simulink model "labFinal_8"  (R2018b)
settings: Solver=FixedStepDiscrete  StartTime=0.0  StopTime=20.0  FixedStep=1  RelTol=1e-3
libraries: hdlsllib x127, simulink_extras x8
(part 1 of 4)
settings Model: Creator=mllax8  LastModifiedBy=mllax8

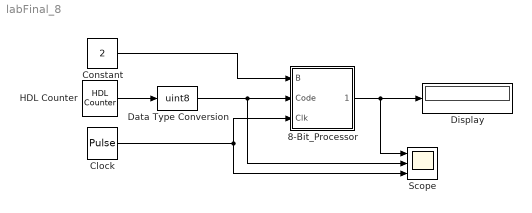
== system labFinal_8 ==
  8-Bit_Processor : Subsystem
  Clock : DiscretePulseGenerator
  Constant : Constant  Value=2  OutDataTypeStr=uint8  SampleTime=1
  Data Type Conversion : DataTypeConversion  OutDataTypeStr=uint8
  Display : Display
  HDL Counter : hdlsllib/Sources/HDL Counter  CountType=Free running  CountInit=0  CountStep=0.5  CountMax=25  CountFromType=Initial value  CountFrom=0  CountResetPort=off  CountLoadPort=off  CountEnbPort=off  CountDirPort=off  CountDataType=Unsigned  CountWordLen=3  CountFracLen=1  CountSampTime=1
      settings: SourceProductBaseCode=HD
  Scope : Scope  NumInputPorts=3
  wires:
  Constant/1 -> 8-Bit_Processor/1(B)
  Clock/1 -> 8-Bit_Processor/3(Clk), Scope/3
  8-Bit_Processor/1(Output) -> Scope/1, Display/1
  Data Type Conversion/1 -> Scope/2, 8-Bit_Processor/2(Code)
  HDL Counter/1 -> Data Type Conversion/1

== system labFinal_8/8-Bit_Processor ==
  B : Inport
  Code : Inport  Port=2
  Clk : Inport  Port=3
  8-bit 4-1 MUX : Subsystem
  8-bit_Adder : Subsystem
  8-bit_Bitwise_AND : Subsystem
  8-bit_Multiply : Subsystem
  8-bit_Register : Subsystem
  8-bit_Subtractor : Subsystem
  Data Type Conversion : DataTypeConversion  OutDataTypeStr=boolean
  Output : Outport
  wires:
  Clk/1 -> Data Type Conversion/1
  Data Type Conversion/1 -> 8-bit_Register/2(Clk)
  Code/1 -> 8-bit 4-1 MUX/1(S)
  8-bit_Adder/1(Sum) -> 8-bit 4-1 MUX/2(x0)
  8-bit_Multiply/1(Product) -> 8-bit 4-1 MUX/3(x1)
  8-bit_Subtractor/1(Diff) -> 8-bit 4-1 MUX/4(x2)
  8-bit_Bitwise_AND/1(Y) -> 8-bit 4-1 MUX/5(x3)
  8-bit_Register/1(Data_Out) -> 8-bit_Bitwise_AND/2(B), 8-bit_Subtractor/1(A), 8-bit_Multiply/2(B), 8-bit_Adder/2(B), Output/1
  8-bit 4-1 MUX/1(Out1) -> 8-bit_Register/1(Data_In)
  B/1 -> 8-bit_Subtractor/2(B), 8-bit_Bitwise_AND/1(A), 8-bit_Multiply/1(A), 8-bit_Adder/1(A)

== system labFinal_8/8-Bit_Processor/8-bit 4-1 MUX ==
  S : Inport
  x0 : Inport  Port=2
  x1 : Inport  Port=3
  x2 : Inport  Port=4
  x3 : Inport  Port=5
  4-1 MUX 2^0 : Subsystem
  4-1 MUX 2^1 : Subsystem
  4-1 MUX 2^2 : Subsystem
  4-1 MUX 2^3 : Subsystem
  4-1 MUX 2^4 : Subsystem
  4-1 MUX 2^5 : Subsystem
  4-1 MUX 2^6 : Subsystem
  4-1 MUX 2^7 : Subsystem
  Concat : Subsystem
  Slicer x0 : Subsystem
  Slicer x1 : Subsystem
  Slicer x2 : Subsystem
  Slicer x3 : Subsystem
  Out1 : Outport
  wires:
  x1/1 -> Slicer x1/1(uint8)
  x0/1 -> Slicer x0/1(uint8)
  4-1 MUX 2^0/1(Z) -> Concat/8(S 2^0)
  Slicer x2/2(B 2^6) -> 4-1 MUX 2^6/4(x2)
  4-1 MUX 2^2/1(Z) -> Concat/6(S 2^2)
  Slicer x2/7(B 2^1) -> 4-1 MUX 2^1/4(x2)
  4-1 MUX 2^5/1(Z) -> Concat/3(S 2^5)
  Slicer x1/3(B 2^5) -> 4-1 MUX 2^5/3(x1)
  Slicer x0/3(B 2^5) -> 4-1 MUX 2^5/2(x0)
  Slicer x3/8("B 2^0 ") -> 4-1 MUX 2^0/5(x3)
  4-1 MUX 2^4/1(Z) -> Concat/4(S 2^4)
  Slicer x2/8("B 2^0 ") -> 4-1 MUX 2^0/4(x2)
  Slicer x3/1(B 2^7) -> 4-1 MUX 2^7/5(x3)
  Slicer x2/4(B 2^4) -> 4-1 MUX 2^4/4(x2)
  Slicer x0/4(B 2^4) -> 4-1 MUX 2^4/2(x0)
  Slicer x1/8("B 2^0 ") -> 4-1 MUX 2^0/3(x1)
  Slicer x3/4(B 2^4) -> 4-1 MUX 2^4/5(x3)
  4-1 MUX 2^3/1(Z) -> Concat/5(S 2^3)
  Slicer x2/3(B 2^5) -> 4-1 MUX 2^5/4(x2)
  Slicer x3/6(B 2^2) -> 4-1 MUX 2^2/5(x3)
  x3/1 -> Slicer x3/1(uint8)
  Slicer x0/6(B 2^2) -> 4-1 MUX 2^2/2(x0)
  4-1 MUX 2^7/1(Z) -> Concat/1(S 2^7)
  Slicer x1/6(B 2^2) -> 4-1 MUX 2^2/3(x1)
  Slicer x3/2(B 2^6) -> 4-1 MUX 2^6/5(x3)
  Slicer x0/7(B 2^1) -> 4-1 MUX 2^1/2(x0)
  Slicer x2/6(B 2^2) -> 4-1 MUX 2^2/4(x2)
  Slicer x3/3(B 2^5) -> 4-1 MUX 2^5/5(x3)
  Slicer x1/7(B 2^1) -> 4-1 MUX 2^1/3(x1)
  x2/1 -> Slicer x2/1(uint8)
  Slicer x0/5(B 2^3) -> 4-1 MUX 2^3/2(x0)
  Slicer x1/5(B 2^3) -> 4-1 MUX 2^3/3(x1)
  Concat/1(unsign Int) -> Out1/1
  Slicer x2/1(B 2^7) -> 4-1 MUX 2^7/4(x2)
  Slicer x0/8("B 2^0 ") -> 4-1 MUX 2^0/2(x0)
  Slicer x2/5(B 2^3) -> 4-1 MUX 2^3/4(x2)
  4-1 MUX 2^1/1(Z) -> Concat/7(S 2^1)
  Slicer x3/7(B 2^1) -> 4-1 MUX 2^1/5(x3)
  4-1 MUX 2^6/1(Z) -> Concat/2(S 2^6)
  Slicer x1/2(B 2^6) -> 4-1 MUX 2^6/3(x1)
  Slicer x1/4(B 2^4) -> 4-1 MUX 2^4/3(x1)
  Slicer x0/2(B 2^6) -> 4-1 MUX 2^6/2(x0)
  Slicer x3/5(B 2^3) -> 4-1 MUX 2^3/5(x3)
  Slicer x1/1(B 2^7) -> 4-1 MUX 2^7/3(x1)
  S/1 -> 4-1 MUX 2^6/1(S), 4-1 MUX 2^5/1(S), 4-1 MUX 2^4/1(S), 4-1 MUX 2^3/1(S), 4-1 MUX 2^2/1(S), 4-1 MUX 2^0/1(S), 4-1 MUX 2^1/1(S), 4-1 MUX 2^7/1(S)
  Slicer x0/1(B 2^7) -> 4-1 MUX 2^7/2(x0)

== system labFinal_8/8-Bit_Processor/8-bit_Adder ==
  A : Inport  OutDataTypeStr=uint8
  B : Inport  Port=2  OutDataTypeStr=uint8
  2^0 : Subsystem
  2^1 : Subsystem
  2^2 : Subsystem
  2^3 : Subsystem
  2^4 : Subsystem
  2^5 : Subsystem
  2^6 : Subsystem
  2^7 : Subsystem
  Concat : Subsystem
  Constant : Constant  Value=0
  Overflow : Constant  Value=-1  OutDataTypeStr=double
  Slicer A : Subsystem
  Slicer B : Subsystem
  Switch : Switch  Criteria=u2 ~= 0
  Sum : Outport
  wires:
  Slicer B/8("B 2^0 ") -> 2^0/2(B)
  2^7/2(Sum) -> Concat/1(S 2^7)
  Slicer B/5(B 2^3) -> 2^3/2(B)
  2^3/2(Sum) -> Concat/5(S 2^3)
  2^5/1(Carry) -> 2^6/3(Carry In)
  Slicer B/4(B 2^4) -> 2^4/2(B)
  Constant/1 -> 2^0/3(Carry In)
  2^4/2(Sum) -> Concat/4(S 2^4)
  Slicer B/6(B 2^2) -> 2^2/2(B)
  2^6/2(Sum) -> Concat/2(S 2^6)
  Slicer A/7(A 2^1) -> 2^1/1(A)
  2^4/1(Carry) -> 2^5/3(Carry In)
  2^5/2(Sum) -> Concat/3(S 2^5)
  2^3/1(Carry) -> 2^4/3(Carry In)
  Slicer B/1(B 2^7) -> 2^7/2(B)
  Slicer A/1(A 2^7) -> 2^7/1(A)
  2^1/1(Carry) -> 2^2/3(Carry In)
  2^0/1(Carry) -> 2^1/3(Carry In)
  Slicer B/3(B 2^5) -> 2^5/2(B)
  Slicer A/8("A 2^0 ") -> 2^0/1(A)
  2^0/2(Sum) -> Concat/8(S 2^0)
  Slicer A/5(A 2^3) -> 2^3/1(A)
  2^2/1(Carry) -> 2^3/3(Carry In)
  Slicer B/7(B 2^1) -> 2^1/2(B)
  Slicer A/4(A 2^4) -> 2^4/1(A)
  2^2/2(Sum) -> Concat/6(S 2^2)
  2^6/1(Carry) -> 2^7/3(Carry In)
  B/1 -> Slicer B/1(uint8)
  Slicer A/2(A 2^6) -> 2^6/1(A)
  2^1/2(Sum) -> Concat/7(S 2^1)
  Slicer A/3(A 2^5) -> 2^5/1(A)
  Slicer B/2(B 2^6) -> 2^6/2(B)
  2^7/1(Carry) -> Switch/2
  Slicer A/6(A 2^2) -> 2^2/1(A)
  A/1 -> Slicer A/1(uint8)
  Overflow/1 -> Switch/1
  Switch/1 -> Sum/1
  Concat/1(unsign Int) -> Switch/3

== system labFinal_8/8-Bit_Processor/8-bit_Bitwise_AND ==
  A : Inport  OutDataTypeStr=uint8
  B : Inport  Port=2  OutDataTypeStr=uint8
  Concat : Subsystem
  Logical Operator{,1..7} (8 alike) : Logic  AllPortsSameDT=off  OutDataTypeStr=boolean
  Slicer A : Subsystem
  Slicer B : Subsystem
  Y : Outport
  wires:
  B/1 -> Slicer B/1(uint8)
  A/1 -> Slicer A/1(uint8)
  Logical Operator/1 -> Concat/8(S 2^0)
  Slicer B/8("B 2^0 ") -> Logical Operator/2
  Slicer A/8("A 2^0 ") -> Logical Operator/1
  Logical Operator1/1 -> Concat/7(S 2^1)
  Logical Operator2/1 -> Concat/6(S 2^2)
  Logical Operator4/1 -> Concat/4(S 2^4)
  Logical Operator3/1 -> Concat/5(S 2^3)
  Logical Operator5/1 -> Concat/3(S 2^5)
  Logical Operator6/1 -> Concat/2(S 2^6)
  Logical Operator7/1 -> Concat/1(S 2^7)
  Slicer B/7(B 2^1) -> Logical Operator1/2
  Slicer B/6(B 2^2) -> Logical Operator2/2
  Slicer B/5(B 2^3) -> Logical Operator3/2
  Slicer B/4(B 2^4) -> Logical Operator4/2
  Slicer B/3(B 2^5) -> Logical Operator5/2
  Slicer B/2(B 2^6) -> Logical Operator6/2
  Slicer B/1(B 2^7) -> Logical Operator7/2
  Slicer A/7(A 2^1) -> Logical Operator1/1
  Slicer A/6(A 2^2) -> Logical Operator2/1
  Slicer A/5(A 2^3) -> Logical Operator3/1
  Slicer A/4(A 2^4) -> Logical Operator4/1
  Slicer A/3(A 2^5) -> Logical Operator5/1
  Slicer A/2(A 2^6) -> Logical Operator6/1
  Slicer A/1(A 2^7) -> Logical Operator7/1
  Concat/1(unsign Int) -> Y/1

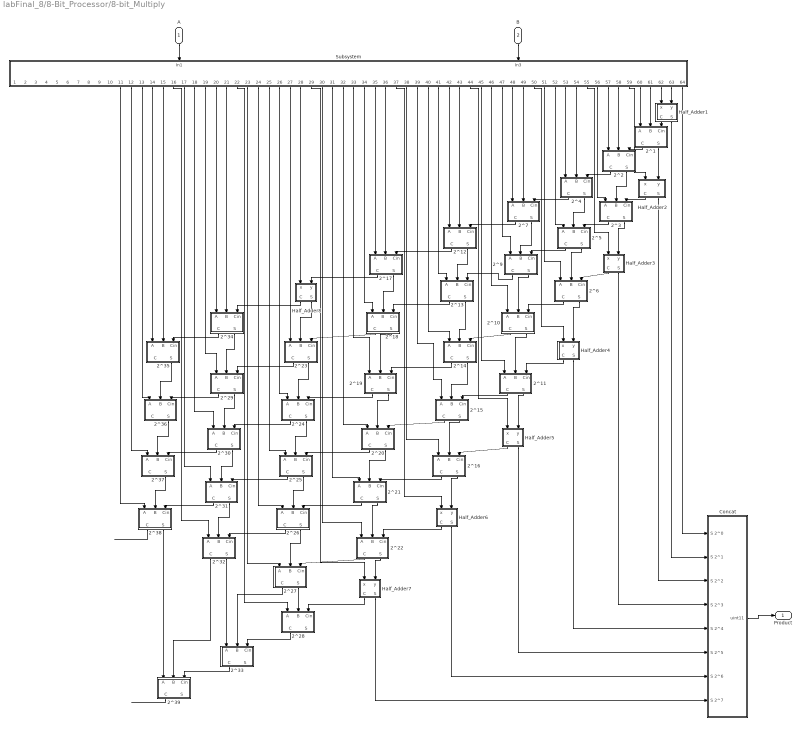
== system labFinal_8/8-Bit_Processor/8-bit_Multiply ==
  A : Inport  OutDataTypeStr=uint8
  B : Inport  Port=2  OutDataTypeStr=uint8
  2^1 : Subsystem
  2^10 : Subsystem
  2^11 : Subsystem
  2^12 : Subsystem
  2^13 : Subsystem
  2^14 : Subsystem
  2^15 : Subsystem
  2^16 : Subsystem
  2^17 : Subsystem
  2^18 : Subsystem
  2^19 : Subsystem
  2^2 : Subsystem
  2^20 : Subsystem
  2^21 : Subsystem
  2^22 : Subsystem
  2^23 : Subsystem
  2^24 : Subsystem
  2^25 : Subsystem
  2^26 : Subsystem
  2^27 : Subsystem
  2^28 : Subsystem
  2^29 : Subsystem
  2^3 : Subsystem
  2^30 : Subsystem
  2^31 : Subsystem
  2^32 : Subsystem
  2^33 : Subsystem
  2^34 : Subsystem
  2^35 : Subsystem
  2^36 : Subsystem
  2^37 : Subsystem
  2^38 : Subsystem
  2^39 : Subsystem
  2^4 : Subsystem
  2^5 : Subsystem
  2^6 : Subsystem
  2^7 : Subsystem
  2^9 : Subsystem
  Concat : Subsystem
  Half_Adder1 : Subsystem
  Half_Adder2 : Subsystem
  Half_Adder3 : Subsystem
  Half_Adder4 : Subsystem
  Half_Adder5 : Subsystem
  Half_Adder6 : Subsystem
  Half_Adder7 : Subsystem
  Half_Adder8 : Subsystem
  Subsystem : Subsystem
  Product : Outport
  wires:
  A/1 -> Subsystem/1(In1)
  B/1 -> Subsystem/2(In3)
  Subsystem/63(A0B1) -> Half_Adder1/2(y)
  Subsystem/62(A1B0) -> Half_Adder1/1(x)
  Half_Adder1/1(C) -> 2^1/3(Cin)
  Subsystem/61(A1B1) -> 2^1/2(B)
  Subsystem/60(A0B2) -> 2^1/1(A)
  Subsystem/59(A2B0) -> Half_Adder2/1(x)
  2^1/2(S) -> Half_Adder2/2(y)
  2^1/1(C) -> 2^2/3(Cin)
  Subsystem/58(A0B3) -> 2^2/2(B)
  Subsystem/57(A1B2) -> 2^2/1(A)
  Half_Adder2/1(C) -> 2^3/3(Cin)
  2^2/2(S) -> 2^3/2(B)
  Subsystem/56(A2B1) -> 2^3/1(A)
  2^3/1(C) -> 2^5/3(Cin)
  Subsystem/55(A3B0) -> Half_Adder3/1(x)
  2^3/2(S) -> Half_Adder3/2(y)
  Subsystem/54(A0B4) -> 2^4/2(B)
  Subsystem/53(A1B3) -> 2^4/1(A)
  2^2/1(C) -> 2^4/3(Cin)
  2^4/1(C) -> 2^7/3(Cin)
  2^4/2(S) -> 2^5/2(B)
  Subsystem/52(A2B2) -> 2^5/1(A)
  2^5/1(C) -> 2^9/3(Cin)
  Half_Adder3/1(C) -> 2^6/3(Cin)
  2^5/2(S) -> 2^6/2(B)
  Subsystem/51(A3B1) -> 2^6/1(A)
  2^6/1(C) -> 2^10/3(Cin)
  2^6/2(S) -> Half_Adder4/2(y)
  Subsystem/50(A4B0) -> Half_Adder4/1(x)
  Half_Adder4/1(C) -> 2^11/3(Cin)
  Subsystem/49(A0B5) -> 2^7/2(B)
  Subsystem/48(A1B4) -> 2^7/1(A)
  Subsystem/47(A2B3) -> 2^9/1(A)
  2^9/2(S) -> 2^10/2(B)
  2^9/1(C) -> 2^13/3(Cin)
  2^7/2(S) -> 2^9/2(B)
  2^7/1(C) -> 2^12/3(Cin)
  Subsystem/46(A3B2) -> 2^10/1(A)
  2^10/1(C) -> 2^14/3(Cin)
  2^10/2(S) -> 2^11/2(B)
  Half_Adder3/2(S) -> Concat/4(S 2^3)
  Half_Adder4/2(S) -> Concat/5(S 2^4)
  2^11/1(C) -> 2^15/3(Cin)
  Subsystem/44(A5B0) -> Half_Adder5/1(x)
  2^11/2(S) -> Half_Adder5/2(y)
  Half_Adder5/2(S) -> Concat/6(S 2^5)
  Half_Adder5/1(C) -> 2^16/3(Cin)
  Subsystem/43(A0B6) -> 2^12/2(B)
  Subsystem/42(A1B5) -> 2^12/1(A)
  2^12/2(S) -> 2^13/2(B)
  Subsystem/41(A2B4) -> 2^13/1(A)
  Subsystem/45(A4B1) -> 2^11/1(A)
  2^13/1(C) -> 2^18/3(Cin)
  2^13/2(S) -> 2^14/2(B)
  Subsystem/40(A3B3) -> 2^14/1(A)
  2^14/2(S) -> 2^15/2(B)
  Subsystem/39(A4B2) -> 2^15/1(A)
  2^15/2(S) -> 2^16/2(B)
  Subsystem/38(A5B1) -> 2^16/1(A)
  2^15/1(C) -> 2^20/3(Cin)
  2^16/1(C) -> 2^21/3(Cin)
  Subsystem/37(A6B0) -> Half_Adder6/1(x)
  2^16/2(S) -> Half_Adder6/2(y)
  Half_Adder6/2(S) -> Concat/7(S 2^6)
  Half_Adder6/1(C) -> 2^22/3(Cin)
  2^17/1(C) -> Half_Adder8/2(y)
  2^12/1(C) -> 2^17/3(Cin)
  2^18/2(S) -> 2^19/2(B)
  2^21/1(C) -> 2^26/3(Cin)
  Subsystem/33(A3B4) -> 2^19/1(A)
  2^19/2(S) -> 2^20/2(B)
  Subsystem/34(A2B5) -> 2^18/1(A)
  Subsystem/32(A4B3) -> 2^20/1(A)
  2^20/2(S) -> 2^21/2(B)
  2^18/1(C) -> 2^23/3(Cin)
  Subsystem/31(A5B2) -> 2^21/1(A)
  2^17/2(S) -> 2^18/2(B)
  Subsystem/36(A0B7) -> 2^17/2(B)
  Subsystem/35(A1B6) -> 2^17/1(A)
  2^14/1(C) -> 2^19/3(Cin)
  2^21/2(S) -> 2^22/2(B)
  Subsystem/30(A6B1) -> 2^22/1(A)
  Subsystem/64(A0B0) -> Concat/1(S 2^0)
  Half_Adder2/2(S) -> Concat/3(S 2^2)
  2^22/2(S) -> Half_Adder7/2(y)
  Subsystem/29(A7B0) -> Half_Adder7/1(x)
  Subsystem/28(A1B7) -> Half_Adder8/1(x)
  Subsystem/27(A2B6) -> 2^23/1(A)
  Half_Adder8/2(S) -> 2^23/2(B)
  Half_Adder8/1(C) -> 2^34/3(Cin)
  2^19/1(C) -> 2^24/3(Cin)
  2^23/2(S) -> 2^24/2(B)
  Subsystem/26(A3B5) -> 2^24/1(A)
  2^20/1(C) -> 2^25/3(Cin)
  2^24/2(S) -> 2^25/2(B)
  Subsystem/25(A4B4) -> 2^25/1(A)
  2^24/1(C) -> 2^30/3(Cin)
  2^25/2(S) -> 2^26/2(B)
  2^25/1(C) -> 2^31/3(Cin)
  2^22/1(C) -> 2^27/3(Cin)
  Subsystem/24(A5B3) -> 2^26/1(A)
  Subsystem/23(A6B2) -> 2^27/1(A)
  Subsystem/22(A7B1) -> 2^28/1(A)
  2^26/2(S) -> 2^27/2(B)
  Half_Adder7/1(C) -> 2^28/3(Cin)
  2^27/2(S) -> 2^28/2(B)
  2^26/1(C) -> 2^32/3(Cin)
  Half_Adder7/2(S) -> Concat/8(S 2^7)
  2^28/1(C) -> 2^33/3(Cin)
  2^29/2(S) -> 2^30/2(B)
  2^30/2(S) -> 2^31/2(B)
  2^31/2(S) -> 2^32/2(B)
  Subsystem/21(A2B7) -> 2^34/2(B)
  Subsystem/20(A3B6) -> 2^34/1(A)
  2^23/1(C) -> 2^29/3(Cin)
  2^34/2(S) -> 2^29/2(B)
  Subsystem/19(A4B5) -> 2^29/1(A)
  Subsystem/18(A5B4) -> 2^30/1(A)
  Subsystem/17(A6B3) -> 2^31/1(A)
  Subsystem/16(A7B2) -> 2^32/1(A)
  2^32/2(S) -> 2^33/1(A)
  2^27/1(C) -> 2^33/2(B)
  2^32/1(C) -> 2^39/2(B)
  2^33/1(C) -> 2^39/3(Cin)
  2^34/1(C) -> 2^35/3(Cin)
  Subsystem/15(A3B7) -> 2^35/2(B)
  Subsystem/14(A4B6) -> 2^35/1(A)
  2^35/2(S) -> 2^36/2(B)
  2^29/1(C) -> 2^36/3(Cin)
  2^30/1(C) -> 2^37/3(Cin)
  2^36/2(S) -> 2^37/2(B)
  Subsystem/13(A5B5) -> 2^36/1(A)
  Subsystem/12(A6B4) -> 2^37/1(A)
  Subsystem/11(A7B3) -> 2^38/1(A)
  2^31/1(C) -> 2^38/3(Cin)
  2^37/2(S) -> 2^38/2(B)
  2^38/2(S) -> 2^39/1(A)
  2^38/1(C) -> ?
  2^39/1(C) -> ?
  Half_Adder1/2(S) -> Concat/2(S 2^1)
  Concat/1(uint11) -> Product/1

== system labFinal_8/8-Bit_Processor/8-bit_Register ==
  Data_In : Inport  OutDataTypeStr=uint8
  Clk : Inport  Port=2
  Concat : Subsystem
  Constant : Constant  OutDataTypeStr=boolean  SampleTime=1
  D Flip-Flop{,1..7} (8 alike) : simulink_extras/Flip Flops/D Flip-Flop
      settings: SourceProductName=Simulink
  Slicer A : Subsystem
  Data_Out : Outport
  wires:
  Data_In/1 -> Slicer A/1(uint8)
  Constant/1 -> D Flip-Flop7/3, D Flip-Flop6/3, D Flip-Flop5/3, D Flip-Flop4/3, D Flip-Flop3/3, D Flip-Flop2/3, D Flip-Flop1/3, D Flip-Flop/3
  Clk/1 -> D Flip-Flop7/2, D Flip-Flop6/2, D Flip-Flop5/2, D Flip-Flop4/2, D Flip-Flop3/2, D Flip-Flop2/2, D Flip-Flop1/2, D Flip-Flop/2
  D Flip-Flop/1 -> Concat/8(S 2^0)
  Slicer A/1(A 2^7) -> D Flip-Flop7/1
  Slicer A/2(A 2^6) -> D Flip-Flop6/1
  Slicer A/3(A 2^5) -> D Flip-Flop5/1
  Slicer A/4(A 2^4) -> D Flip-Flop4/1
  Slicer A/5(A 2^3) -> D Flip-Flop3/1
  Slicer A/6(A 2^2) -> D Flip-Flop2/1
  Slicer A/7(A 2^1) -> D Flip-Flop1/1
  Slicer A/8("A 2^0 ") -> D Flip-Flop/1
  D Flip-Flop1/1 -> Concat/7(S 2^1)
  D Flip-Flop7/1 -> Concat/1(S 2^7)
  D Flip-Flop6/1 -> Concat/2(S 2^6)
  D Flip-Flop5/1 -> Concat/3(S 2^5)
  D Flip-Flop4/1 -> Concat/4(S 2^4)
  D Flip-Flop3/1 -> Concat/5(S 2^3)
  D Flip-Flop2/1 -> Concat/6(S 2^2)
  Concat/1(unsign Int) -> Data_Out/1

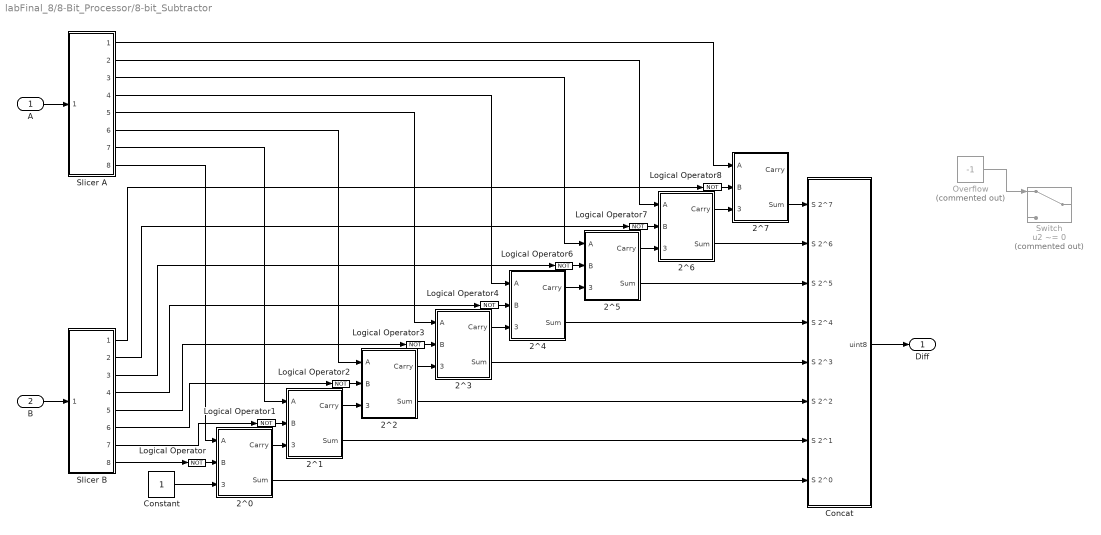
== system labFinal_8/8-Bit_Processor/8-bit_Subtractor ==
  A : Inport  OutDataTypeStr=uint8
  B : Inport  Port=2  OutDataTypeStr=uint8
  2^0 : Subsystem
  2^1 : Subsystem
  2^2 : Subsystem
  2^3 : Subsystem
  2^4 : Subsystem
  2^5 : Subsystem
  2^6 : Subsystem
  2^7 : Subsystem
  Concat : Subsystem
  Constant : Constant  SampleTime=1
  Logical Operator{,1..4,6..8} (8 alike) : Logic  Operator=NOT  AllPortsSameDT=off  OutDataTypeStr=boolean
  Overflow : Constant  Commented=on  Value=-1  OutDataTypeStr=double
  Slicer A : Subsystem
  Slicer B : Subsystem
  Switch : Switch  Commented=on  Criteria=u2 ~= 0
  Diff : Outport
  wires:
  2^7/2(Sum) -> Concat/1(S 2^7)
  Slicer B/5(B 2^3) -> Logical Operator3/1
  2^3/2(Sum) -> Concat/5(S 2^3)
  2^5/1(Carry) -> 2^6/3(Carry In)
  Slicer B/4(B 2^4) -> Logical Operator4/1
  Constant/1 -> 2^0/3(Carry In)
  2^4/2(Sum) -> Concat/4(S 2^4)
  Slicer B/6(B 2^2) -> Logical Operator2/1
  2^6/2(Sum) -> Concat/2(S 2^6)
  Slicer A/7(A 2^1) -> 2^1/1(A)
  2^4/1(Carry) -> 2^5/3(Carry In)
  2^5/2(Sum) -> Concat/3(S 2^5)
  2^3/1(Carry) -> 2^4/3(Carry In)
  Slicer B/1(B 2^7) -> Logical Operator8/1
  Slicer A/1(A 2^7) -> 2^7/1(A)
  2^1/1(Carry) -> 2^2/3(Carry In)
  2^0/1(Carry) -> 2^1/3(Carry In)
  Slicer B/3(B 2^5) -> Logical Operator6/1
  Slicer A/8("A 2^0 ") -> 2^0/1(A)
  2^0/2(Sum) -> Concat/8(S 2^0)
  Slicer A/5(A 2^3) -> 2^3/1(A)
  2^2/1(Carry) -> 2^3/3(Carry In)
  Slicer B/7(B 2^1) -> Logical Operator1/1
  Slicer A/4(A 2^4) -> 2^4/1(A)
  2^2/2(Sum) -> Concat/6(S 2^2)
  2^6/1(Carry) -> 2^7/3(Carry In)
  B/1 -> Slicer B/1(uint8)
  Slicer A/2(A 2^6) -> 2^6/1(A)
  2^1/2(Sum) -> Concat/7(S 2^1)
  Slicer A/3(A 2^5) -> 2^5/1(A)
  Slicer B/2(B 2^6) -> Logical Operator7/1
  Slicer A/6(A 2^2) -> 2^2/1(A)
  A/1 -> Slicer A/1(uint8)
  Overflow/1 -> Switch/1
  Logical Operator/1 -> 2^0/2(B)
  Slicer B/8("B 2^0 ") -> Logical Operator/1
  Logical Operator1/1 -> 2^1/2(B)
  Logical Operator2/1 -> 2^2/2(B)
  Logical Operator3/1 -> 2^3/2(B)
  Logical Operator4/1 -> 2^4/2(B)
  Logical Operator6/1 -> 2^5/2(B)
  Logical Operator7/1 -> 2^6/2(B)
  Logical Operator8/1 -> 2^7/2(B)
  Concat/1(uint8) -> Diff/1

== system labFinal_8/8-Bit_Processor/8-bit 4-1 MUX/4-1 MUX 2^0 ==
  S : Inport  OutDataTypeStr=uint8
  x0 : Inport  Port=2  OutDataTypeStr=boolean
  x1 : Inport  Port=3  OutDataTypeStr=boolean
  x2 : Inport  Port=4  OutDataTypeStr=boolean
  x3 : Inport  Port=5  OutDataTypeStr=boolean
  2-1 MUX1 : Subsystem
  2-1 MUX2 : Subsystem
  2-1 MUX3 : Subsystem
  Slicer Code : Subsystem
  Z : Outport
  wires:
  Slicer Code/2("S 2^0 ") -> 2-1 MUX3/1(S), 2-1 MUX1/1(S)
  x0/1 -> 2-1 MUX3/2(I0)
  x1/1 -> 2-1 MUX3/3(I1)
  x2/1 -> 2-1 MUX1/2(I0)
  x3/1 -> 2-1 MUX1/3(I1)
  2-1 MUX3/1(Z) -> 2-1 MUX2/2(I0)
  2-1 MUX1/1(Z) -> 2-1 MUX2/3(I1)
  2-1 MUX2/1(Z) -> Z/1
  S/1 -> Slicer Code/1(uint8)
  Slicer Code/1(S 2^1) -> 2-1 MUX2/1(S)

== system labFinal_8/8-Bit_Processor/8-bit 4-1 MUX/4-1 MUX 2^1 ==
  S : Inport  OutDataTypeStr=uint8
  x0 : Inport  Port=2  OutDataTypeStr=boolean
  x1 : Inport  Port=3  OutDataTypeStr=boolean
  x2 : Inport  Port=4  OutDataTypeStr=boolean
  x3 : Inport  Port=5  OutDataTypeStr=boolean
  2-1 MUX1 : Subsystem
  2-1 MUX2 : Subsystem
  2-1 MUX3 : Subsystem
  Slicer Code : Subsystem
  Z : Outport
  wires:
  Slicer Code/2("S 2^0 ") -> 2-1 MUX3/1(S), 2-1 MUX1/1(S)
  x0/1 -> 2-1 MUX3/2(I0)
  x1/1 -> 2-1 MUX3/3(I1)
  x2/1 -> 2-1 MUX1/2(I0)
  x3/1 -> 2-1 MUX1/3(I1)
  2-1 MUX3/1(Z) -> 2-1 MUX2/2(I0)
  2-1 MUX1/1(Z) -> 2-1 MUX2/3(I1)
  2-1 MUX2/1(Z) -> Z/1
  S/1 -> Slicer Code/1(uint8)
  Slicer Code/1(S 2^1) -> 2-1 MUX2/1(S)

== system labFinal_8/8-Bit_Processor/8-bit 4-1 MUX/4-1 MUX 2^2 ==
  S : Inport  OutDataTypeStr=uint8
  x0 : Inport  Port=2  OutDataTypeStr=boolean
  x1 : Inport  Port=3  OutDataTypeStr=boolean
  x2 : Inport  Port=4  OutDataTypeStr=boolean
  x3 : Inport  Port=5  OutDataTypeStr=boolean
  2-1 MUX1 : Subsystem
  2-1 MUX2 : Subsystem
  2-1 MUX3 : Subsystem
  Slicer Code : Subsystem
  Z : Outport
  wires:
  Slicer Code/2("S 2^0 ") -> 2-1 MUX3/1(S), 2-1 MUX1/1(S)
  x0/1 -> 2-1 MUX3/2(I0)
  x1/1 -> 2-1 MUX3/3(I1)
  x2/1 -> 2-1 MUX1/2(I0)
  x3/1 -> 2-1 MUX1/3(I1)
  2-1 MUX3/1(Z) -> 2-1 MUX2/2(I0)
  2-1 MUX1/1(Z) -> 2-1 MUX2/3(I1)
  2-1 MUX2/1(Z) -> Z/1
  S/1 -> Slicer Code/1(uint8)
  Slicer Code/1(S 2^1) -> 2-1 MUX2/1(S)

== system labFinal_8/8-Bit_Processor/8-bit 4-1 MUX/4-1 MUX 2^3 ==
  S : Inport  OutDataTypeStr=uint8
  x0 : Inport  Port=2  OutDataTypeStr=boolean
  x1 : Inport  Port=3  OutDataTypeStr=boolean
  x2 : Inport  Port=4  OutDataTypeStr=boolean
  x3 : Inport  Port=5  OutDataTypeStr=boolean
  2-1 MUX1 : Subsystem
  2-1 MUX2 : Subsystem
  2-1 MUX3 : Subsystem
  Slicer Code : Subsystem
  Z : Outport
  wires:
  Slicer Code/2("S 2^0 ") -> 2-1 MUX3/1(S), 2-1 MUX1/1(S)
  x0/1 -> 2-1 MUX3/2(I0)
  x1/1 -> 2-1 MUX3/3(I1)
  x2/1 -> 2-1 MUX1/2(I0)
  x3/1 -> 2-1 MUX1/3(I1)
  2-1 MUX3/1(Z) -> 2-1 MUX2/2(I0)
  2-1 MUX1/1(Z) -> 2-1 MUX2/3(I1)
  2-1 MUX2/1(Z) -> Z/1
  S/1 -> Slicer Code/1(uint8)
  Slicer Code/1(S 2^1) -> 2-1 MUX2/1(S)

== system labFinal_8/8-Bit_Processor/8-bit 4-1 MUX/4-1 MUX 2^4 ==
  S : Inport  OutDataTypeStr=uint8
  x0 : Inport  Port=2  OutDataTypeStr=boolean
  x1 : Inport  Port=3  OutDataTypeStr=boolean
  x2 : Inport  Port=4  OutDataTypeStr=boolean
  x3 : Inport  Port=5  OutDataTypeStr=boolean
  2-1 MUX1 : Subsystem
  2-1 MUX2 : Subsystem
  2-1 MUX3 : Subsystem
  Slicer Code : Subsystem
  Z : Outport
  wires:
  Slicer Code/2("S 2^0 ") -> 2-1 MUX3/1(S), 2-1 MUX1/1(S)
  x0/1 -> 2-1 MUX3/2(I0)
  x1/1 -> 2-1 MUX3/3(I1)
  x2/1 -> 2-1 MUX1/2(I0)
  x3/1 -> 2-1 MUX1/3(I1)
  2-1 MUX3/1(Z) -> 2-1 MUX2/2(I0)
  2-1 MUX1/1(Z) -> 2-1 MUX2/3(I1)
  2-1 MUX2/1(Z) -> Z/1
  S/1 -> Slicer Code/1(uint8)
  Slicer Code/1(S 2^1) -> 2-1 MUX2/1(S)

== system labFinal_8/8-Bit_Processor/8-bit 4-1 MUX/4-1 MUX 2^5 ==
  S : Inport  OutDataTypeStr=uint8
  x0 : Inport  Port=2  OutDataTypeStr=boolean
  x1 : Inport  Port=3  OutDataTypeStr=boolean
  x2 : Inport  Port=4  OutDataTypeStr=boolean
  x3 : Inport  Port=5  OutDataTypeStr=boolean
  2-1 MUX1 : Subsystem
  2-1 MUX2 : Subsystem
  2-1 MUX3 : Subsystem
  Slicer Code : Subsystem
  Z : Outport
  wires:
  Slicer Code/2("S 2^0 ") -> 2-1 MUX3/1(S), 2-1 MUX1/1(S)
  x0/1 -> 2-1 MUX3/2(I0)
  x1/1 -> 2-1 MUX3/3(I1)
  x2/1 -> 2-1 MUX1/2(I0)
  x3/1 -> 2-1 MUX1/3(I1)
  2-1 MUX3/1(Z) -> 2-1 MUX2/2(I0)
  2-1 MUX1/1(Z) -> 2-1 MUX2/3(I1)
  2-1 MUX2/1(Z) -> Z/1
  S/1 -> Slicer Code/1(uint8)
  Slicer Code/1(S 2^1) -> 2-1 MUX2/1(S)

== system labFinal_8/8-Bit_Processor/8-bit 4-1 MUX/4-1 MUX 2^6 ==
  S : Inport  OutDataTypeStr=uint8
  x0 : Inport  Port=2  OutDataTypeStr=boolean
  x1 : Inport  Port=3  OutDataTypeStr=boolean
  x2 : Inport  Port=4  OutDataTypeStr=boolean
  x3 : Inport  Port=5  OutDataTypeStr=boolean
  2-1 MUX1 : Subsystem
  2-1 MUX2 : Subsystem
  2-1 MUX3 : Subsystem
  Slicer Code : Subsystem
  Z : Outport
  wires:
  Slicer Code/2("S 2^0 ") -> 2-1 MUX3/1(S), 2-1 MUX1/1(S)
  x0/1 -> 2-1 MUX3/2(I0)
  x1/1 -> 2-1 MUX3/3(I1)
  x2/1 -> 2-1 MUX1/2(I0)
  x3/1 -> 2-1 MUX1/3(I1)
  2-1 MUX3/1(Z) -> 2-1 MUX2/2(I0)
  2-1 MUX1/1(Z) -> 2-1 MUX2/3(I1)
  2-1 MUX2/1(Z) -> Z/1
  S/1 -> Slicer Code/1(uint8)
  Slicer Code/1(S 2^1) -> 2-1 MUX2/1(S)

== system labFinal_8/8-Bit_Processor/8-bit 4-1 MUX/4-1 MUX 2^7 ==
  S : Inport  OutDataTypeStr=uint8
  x0 : Inport  Port=2  OutDataTypeStr=boolean
  x1 : Inport  Port=3  OutDataTypeStr=boolean
  x2 : Inport  Port=4  OutDataTypeStr=boolean
  x3 : Inport  Port=5  OutDataTypeStr=boolean
  2-1 MUX1 : Subsystem
  2-1 MUX2 : Subsystem
  2-1 MUX3 : Subsystem
  Slicer Code : Subsystem
  Z : Outport
  wires:
  Slicer Code/2("S 2^0 ") -> 2-1 MUX3/1(S), 2-1 MUX1/1(S)
  x0/1 -> 2-1 MUX3/2(I0)
  x1/1 -> 2-1 MUX3/3(I1)
  x2/1 -> 2-1 MUX1/2(I0)
  x3/1 -> 2-1 MUX1/3(I1)
  2-1 MUX3/1(Z) -> 2-1 MUX2/2(I0)
  2-1 MUX1/1(Z) -> 2-1 MUX2/3(I1)
  2-1 MUX2/1(Z) -> Z/1
  S/1 -> Slicer Code/1(uint8)
  Slicer Code/1(S 2^1) -> 2-1 MUX2/1(S)

== system labFinal_8/8-Bit_Processor/8-bit 4-1 MUX/Concat ==
  S 2^7 : Inport
  S 2^6 : Inport  Port=2
  S 2^5 : Inport  Port=3
  S 2^4 : Inport  Port=4
  S 2^3 : Inport  Port=5
  S 2^2 : Inport  Port=6
  S 2^1 : Inport  Port=7
  S 2^0 : Inport  Port=8
  Bit Concat : hdlsllib/Logic and Bit Operations/Bit Concat  numInputs=8
      settings: SourceProductName=HDL Coder  SourceProductBaseCode=HD
  unsign Int : Outport
  wires:
  Bit Concat/1 -> unsign Int/1
  S 2^3/1 -> Bit Concat/5
  S 2^5/1 -> Bit Concat/3
  S 2^4/1 -> Bit Concat/4
  S 2^0/1 -> Bit Concat/8
  S 2^7/1 -> Bit Concat/1
  S 2^1/1 -> Bit Concat/7
  S 2^6/1 -> Bit Concat/2
  S 2^2/1 -> Bit Concat/6

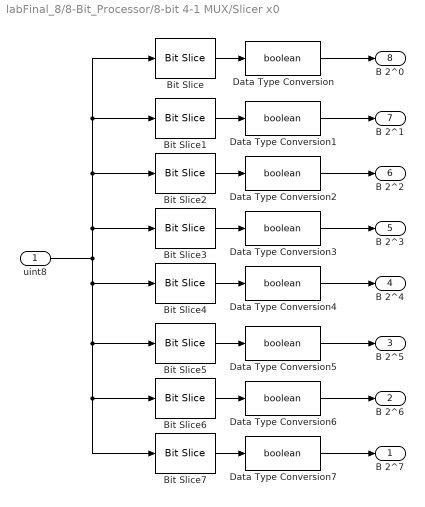
== system labFinal_8/8-Bit_Processor/8-bit 4-1 MUX/Slicer x0 ==
  uint8 : Inport  OutDataTypeStr=uint8  SampleTime=1
  Bit Slice : hdlsllib/Logic and Bit Operations/Bit Slice  lidx=0  ridx=0
  Bit Slice1 : hdlsllib/Logic and Bit Operations/Bit Slice  lidx=1  ridx=1
  Bit Slice2 : hdlsllib/Logic and Bit Operations/Bit Slice  lidx=2  ridx=2
  Bit Slice3 : hdlsllib/Logic and Bit Operations/Bit Slice  lidx=3  ridx=3
  Bit Slice4 : hdlsllib/Logic and Bit Operations/Bit Slice  lidx=4  ridx=4
  Bit Slice5 : hdlsllib/Logic and Bit Operations/Bit Slice  lidx=5  ridx=5
  Bit Slice6 : hdlsllib/Logic and Bit Operations/Bit Slice  lidx=6  ridx=6
  Bit Slice7 : hdlsllib/Logic and Bit Operations/Bit Slice  lidx=7  ridx=7
  Data Type Conversion{,1..7} (8 alike) : DataTypeConversion  OutDataTypeStr=boolean
  B 2^7 : Outport
  B 2^6 : Outport  Port=2
  B 2^5 : Outport  Port=3
  B 2^4 : Outport  Port=4
  B 2^3 : Outport  Port=5
  B 2^2 : Outport  Port=6
  B 2^1 : Outport  Port=7
  "B 2^0 " : Outport  Port=8
  wires:
  Data Type Conversion/1 -> "B 2^0 "/1
  Data Type Conversion5/1 -> B 2^5/1
  Bit Slice1/1 -> Data Type Conversion1/1
  Bit Slice5/1 -> Data Type Conversion5/1
  Bit Slice7/1 -> Data Type Conversion7/1
  Bit Slice2/1 -> Data Type Conversion2/1
  Bit Slice3/1 -> Data Type Conversion3/1
  Data Type Conversion6/1 -> B 2^6/1
  Bit Slice4/1 -> Data Type Conversion4/1
  uint8/1 -> Bit Slice4/1, Bit Slice5/1, Bit Slice6/1, Bit Slice7/1, Bit Slice3/1, Bit Slice2/1, Bit Slice1/1, Bit Slice/1
  Data Type Conversion1/1 -> B 2^1/1
  Data Type Conversion2/1 -> B 2^2/1
  Bit Slice/1 -> Data Type Conversion/1
  Bit Slice6/1 -> Data Type Conversion6/1
  Data Type Conversion3/1 -> B 2^3/1
  Data Type Conversion4/1 -> B 2^4/1
  Data Type Conversion7/1 -> B 2^7/1

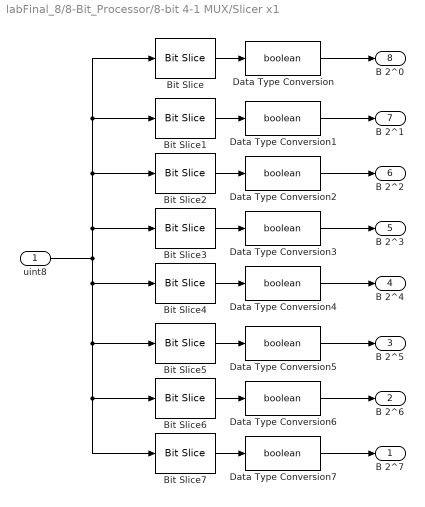
== system labFinal_8/8-Bit_Processor/8-bit 4-1 MUX/Slicer x1 ==
  uint8 : Inport  OutDataTypeStr=uint8  SampleTime=1
  Bit Slice : hdlsllib/Logic and Bit Operations/Bit Slice  lidx=0  ridx=0
  Bit Slice1 : hdlsllib/Logic and Bit Operations/Bit Slice  lidx=1  ridx=1
  Bit Slice2 : hdlsllib/Logic and Bit Operations/Bit Slice  lidx=2  ridx=2
  Bit Slice3 : hdlsllib/Logic and Bit Operations/Bit Slice  lidx=3  ridx=3
  Bit Slice4 : hdlsllib/Logic and Bit Operations/Bit Slice  lidx=4  ridx=4
  Bit Slice5 : hdlsllib/Logic and Bit Operations/Bit Slice  lidx=5  ridx=5
  Bit Slice6 : hdlsllib/Logic and Bit Operations/Bit Slice  lidx=6  ridx=6
  Bit Slice7 : hdlsllib/Logic and Bit Operations/Bit Slice  lidx=7  ridx=7
  Data Type Conversion{,1..7} (8 alike) : DataTypeConversion  OutDataTypeStr=boolean
  B 2^7 : Outport
  B 2^6 : Outport  Port=2
  B 2^5 : Outport  Port=3
  B 2^4 : Outport  Port=4
  B 2^3 : Outport  Port=5
  B 2^2 : Outport  Port=6
  B 2^1 : Outport  Port=7
  "B 2^0 " : Outport  Port=8
  wires:
  Data Type Conversion/1 -> "B 2^0 "/1
  Data Type Conversion5/1 -> B 2^5/1
  Bit Slice1/1 -> Data Type Conversion1/1
  Bit Slice5/1 -> Data Type Conversion5/1
  Bit Slice7/1 -> Data Type Conversion7/1
  Bit Slice2/1 -> Data Type Conversion2/1
  Bit Slice3/1 -> Data Type Conversion3/1
  Data Type Conversion6/1 -> B 2^6/1
  Bit Slice4/1 -> Data Type Conversion4/1
  uint8/1 -> Bit Slice4/1, Bit Slice5/1, Bit Slice6/1, Bit Slice7/1, Bit Slice3/1, Bit Slice2/1, Bit Slice1/1, Bit Slice/1
  Data Type Conversion1/1 -> B 2^1/1
  Data Type Conversion2/1 -> B 2^2/1
  Bit Slice/1 -> Data Type Conversion/1
  Bit Slice6/1 -> Data Type Conversion6/1
  Data Type Conversion3/1 -> B 2^3/1
  Data Type Conversion4/1 -> B 2^4/1
  Data Type Conversion7/1 -> B 2^7/1

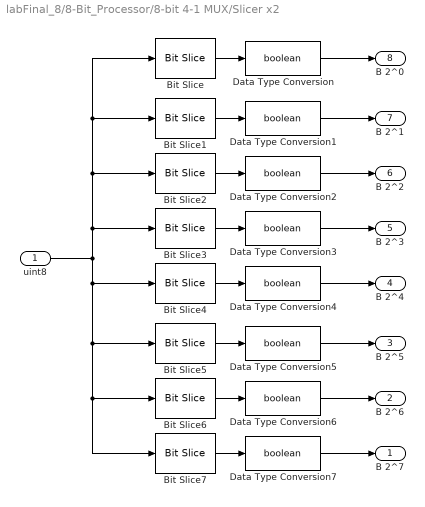
== system labFinal_8/8-Bit_Processor/8-bit 4-1 MUX/Slicer x2 ==
  uint8 : Inport  OutDataTypeStr=uint8  SampleTime=1
  Bit Slice : hdlsllib/Logic and Bit Operations/Bit Slice  lidx=0  ridx=0
  Bit Slice1 : hdlsllib/Logic and Bit Operations/Bit Slice  lidx=1  ridx=1
  Bit Slice2 : hdlsllib/Logic and Bit Operations/Bit Slice  lidx=2  ridx=2
  Bit Slice3 : hdlsllib/Logic and Bit Operations/Bit Slice  lidx=3  ridx=3
  Bit Slice4 : hdlsllib/Logic and Bit Operations/Bit Slice  lidx=4  ridx=4
  Bit Slice5 : hdlsllib/Logic and Bit Operations/Bit Slice  lidx=5  ridx=5
  Bit Slice6 : hdlsllib/Logic and Bit Operations/Bit Slice  lidx=6  ridx=6
  Bit Slice7 : hdlsllib/Logic and Bit Operations/Bit Slice  lidx=7  ridx=7
  Data Type Conversion{,1..7} (8 alike) : DataTypeConversion  OutDataTypeStr=boolean
  B 2^7 : Outport
  B 2^6 : Outport  Port=2
  B 2^5 : Outport  Port=3
  B 2^4 : Outport  Port=4
  B 2^3 : Outport  Port=5
  B 2^2 : Outport  Port=6
  B 2^1 : Outport  Port=7
  "B 2^0 " : Outport  Port=8
  wires:
  Data Type Conversion/1 -> "B 2^0 "/1
  Data Type Conversion5/1 -> B 2^5/1
  Bit Slice1/1 -> Data Type Conversion1/1
  Bit Slice5/1 -> Data Type Conversion5/1
  Bit Slice7/1 -> Data Type Conversion7/1
  Bit Slice2/1 -> Data Type Conversion2/1
  Bit Slice3/1 -> Data Type Conversion3/1
  Data Type Conversion6/1 -> B 2^6/1
  Bit Slice4/1 -> Data Type Conversion4/1
  uint8/1 -> Bit Slice4/1, Bit Slice5/1, Bit Slice6/1, Bit Slice7/1, Bit Slice3/1, Bit Slice2/1, Bit Slice1/1, Bit Slice/1
  Data Type Conversion1/1 -> B 2^1/1
  Data Type Conversion2/1 -> B 2^2/1
  Bit Slice/1 -> Data Type Conversion/1
  Bit Slice6/1 -> Data Type Conversion6/1
  Data Type Conversion3/1 -> B 2^3/1
  Data Type Conversion4/1 -> B 2^4/1
  Data Type Conversion7/1 -> B 2^7/1

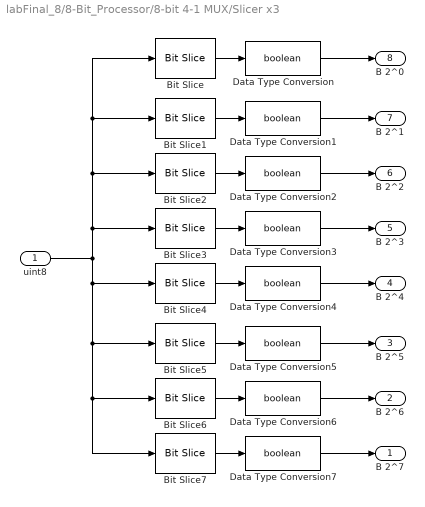
== system labFinal_8/8-Bit_Processor/8-bit 4-1 MUX/Slicer x3 ==
  uint8 : Inport  OutDataTypeStr=uint8  SampleTime=1
  Bit Slice : hdlsllib/Logic and Bit Operations/Bit Slice  lidx=0  ridx=0
  Bit Slice1 : hdlsllib/Logic and Bit Operations/Bit Slice  lidx=1  ridx=1
  Bit Slice2 : hdlsllib/Logic and Bit Operations/Bit Slice  lidx=2  ridx=2
  Bit Slice3 : hdlsllib/Logic and Bit Operations/Bit Slice  lidx=3  ridx=3
  Bit Slice4 : hdlsllib/Logic and Bit Operations/Bit Slice  lidx=4  ridx=4
  Bit Slice5 : hdlsllib/Logic and Bit Operations/Bit Slice  lidx=5  ridx=5
  Bit Slice6 : hdlsllib/Logic and Bit Operations/Bit Slice  lidx=6  ridx=6
  Bit Slice7 : hdlsllib/Logic and Bit Operations/Bit Slice  lidx=7  ridx=7
  Data Type Conversion{,1..7} (8 alike) : DataTypeConversion  OutDataTypeStr=boolean
  B 2^7 : Outport
  B 2^6 : Outport  Port=2
  B 2^5 : Outport  Port=3
  B 2^4 : Outport  Port=4
  B 2^3 : Outport  Port=5
  B 2^2 : Outport  Port=6
  B 2^1 : Outport  Port=7
  "B 2^0 " : Outport  Port=8
  wires:
  Data Type Conversion/1 -> "B 2^0 "/1
  Data Type Conversion5/1 -> B 2^5/1
  Bit Slice1/1 -> Data Type Conversion1/1
  Bit Slice5/1 -> Data Type Conversion5/1
  Bit Slice7/1 -> Data Type Conversion7/1
  Bit Slice2/1 -> Data Type Conversion2/1
  Bit Slice3/1 -> Data Type Conversion3/1
  Data Type Conversion6/1 -> B 2^6/1
  Bit Slice4/1 -> Data Type Conversion4/1
  uint8/1 -> Bit Slice4/1, Bit Slice5/1, Bit Slice6/1, Bit Slice7/1, Bit Slice3/1, Bit Slice2/1, Bit Slice1/1, Bit Slice/1
  Data Type Conversion1/1 -> B 2^1/1
  Data Type Conversion2/1 -> B 2^2/1
  Bit Slice/1 -> Data Type Conversion/1
  Bit Slice6/1 -> Data Type Conversion6/1
  Data Type Conversion3/1 -> B 2^3/1
  Data Type Conversion4/1 -> B 2^4/1
  Data Type Conversion7/1 -> B 2^7/1

== system labFinal_8/8-Bit_Processor/8-bit_Adder/2^0 ==
  A : Inport
  B : Inport  Port=2
  Carry In : Inport  Port=3
  Half_Adder : Subsystem
  Half_Adder1 : Subsystem
  Logical Operator : Logic  Operator=OR  AllPortsSameDT=off  OutDataTypeStr=boolean
  Carry : Outport
  Sum : Outport  Port=2
  wires:
  Half_Adder1/1(Sum) -> Sum/1
  Carry In/1 -> Half_Adder1/2(y)
  Logical Operator/1 -> Carry/1
  Half_Adder1/2(Carry) -> Logical Operator/1
  A/1 -> Half_Adder/1(x)
  B/1 -> Half_Adder/2(y)
  Half_Adder/2(Carry) -> Logical Operator/2
  Half_Adder/1(Sum) -> Half_Adder1/1(x)

== system labFinal_8/8-Bit_Processor/8-bit_Adder/2^1 ==
  A : Inport
  B : Inport  Port=2
  Carry In : Inport  Port=3
  Half_Adder : Subsystem
  Half_Adder1 : Subsystem
  Logical Operator : Logic  Operator=OR  AllPortsSameDT=off  OutDataTypeStr=boolean
  Carry : Outport
  Sum : Outport  Port=2
  wires:
  Half_Adder1/1(Sum) -> Sum/1
  Carry In/1 -> Half_Adder1/2(y)
  Logical Operator/1 -> Carry/1
  Half_Adder1/2(Carry) -> Logical Operator/1
  A/1 -> Half_Adder/1(x)
  B/1 -> Half_Adder/2(y)
  Half_Adder/2(Carry) -> Logical Operator/2
  Half_Adder/1(Sum) -> Half_Adder1/1(x)

== system labFinal_8/8-Bit_Processor/8-bit_Adder/2^2 ==
  A : Inport
  B : Inport  Port=2
  Carry In : Inport  Port=3
  Half_Adder : Subsystem
  Half_Adder1 : Subsystem
  Logical Operator : Logic  Operator=OR  AllPortsSameDT=off  OutDataTypeStr=boolean
  Carry : Outport
  Sum : Outport  Port=2
  wires:
  Half_Adder1/1(Sum) -> Sum/1
  Carry In/1 -> Half_Adder1/2(y)
  Logical Operator/1 -> Carry/1
  Half_Adder1/2(Carry) -> Logical Operator/1
  A/1 -> Half_Adder/1(x)
  B/1 -> Half_Adder/2(y)
  Half_Adder/2(Carry) -> Logical Operator/2
  Half_Adder/1(Sum) -> Half_Adder1/1(x)

== system labFinal_8/8-Bit_Processor/8-bit_Adder/2^3 ==
  A : Inport
  B : Inport  Port=2
  Carry In : Inport  Port=3
  Half_Adder : Subsystem
  Half_Adder1 : Subsystem
  Logical Operator : Logic  Operator=OR  AllPortsSameDT=off  OutDataTypeStr=boolean
  Carry : Outport
  Sum : Outport  Port=2
  wires:
  Half_Adder1/1(Sum) -> Sum/1
  Carry In/1 -> Half_Adder1/2(y)
  Logical Operator/1 -> Carry/1
  Half_Adder1/2(Carry) -> Logical Operator/1
  A/1 -> Half_Adder/1(x)
  B/1 -> Half_Adder/2(y)
  Half_Adder/2(Carry) -> Logical Operator/2
  Half_Adder/1(Sum) -> Half_Adder1/1(x)

== system labFinal_8/8-Bit_Processor/8-bit_Adder/2^4 ==
  A : Inport
  B : Inport  Port=2
  Carry In : Inport  Port=3
  Half_Adder : Subsystem
  Half_Adder1 : Subsystem
  Logical Operator : Logic  Operator=OR  AllPortsSameDT=off  OutDataTypeStr=boolean
  Carry : Outport
  Sum : Outport  Port=2
  wires:
  Half_Adder1/1(Sum) -> Sum/1
  Carry In/1 -> Half_Adder1/2(y)
  Logical Operator/1 -> Carry/1
  Half_Adder1/2(Carry) -> Logical Operator/1
  A/1 -> Half_Adder/1(x)
  B/1 -> Half_Adder/2(y)
  Half_Adder/2(Carry) -> Logical Operator/2
  Half_Adder/1(Sum) -> Half_Adder1/1(x)

== system labFinal_8/8-Bit_Processor/8-bit_Adder/2^5 ==
  A : Inport
  B : Inport  Port=2
  Carry In : Inport  Port=3
  Half_Adder : Subsystem
  Half_Adder1 : Subsystem
  Logical Operator : Logic  Operator=OR  AllPortsSameDT=off  OutDataTypeStr=boolean
  Carry : Outport
  Sum : Outport  Port=2
  wires:
  Half_Adder1/1(Sum) -> Sum/1
  Carry In/1 -> Half_Adder1/2(y)
  Logical Operator/1 -> Carry/1
  Half_Adder1/2(Carry) -> Logical Operator/1
  A/1 -> Half_Adder/1(x)
  B/1 -> Half_Adder/2(y)
  Half_Adder/2(Carry) -> Logical Operator/2
  Half_Adder/1(Sum) -> Half_Adder1/1(x)

== system labFinal_8/8-Bit_Processor/8-bit_Adder/2^6 ==
  A : Inport
  B : Inport  Port=2
  Carry In : Inport  Port=3
  Half_Adder : Subsystem
  Half_Adder1 : Subsystem
  Logical Operator : Logic  Operator=OR  AllPortsSameDT=off  OutDataTypeStr=boolean
  Carry : Outport
  Sum : Outport  Port=2
  wires:
  Half_Adder1/1(Sum) -> Sum/1
  Carry In/1 -> Half_Adder1/2(y)
  Logical Operator/1 -> Carry/1
  Half_Adder1/2(Carry) -> Logical Operator/1
  A/1 -> Half_Adder/1(x)
  B/1 -> Half_Adder/2(y)
  Half_Adder/2(Carry) -> Logical Operator/2
  Half_Adder/1(Sum) -> Half_Adder1/1(x)

== system labFinal_8/8-Bit_Processor/8-bit_Adder/2^7 ==
  A : Inport
  B : Inport  Port=2
  Carry In : Inport  Port=3
  Half_Adder : Subsystem
  Half_Adder1 : Subsystem
  Logical Operator : Logic  Operator=OR  AllPortsSameDT=off  OutDataTypeStr=boolean
  Carry : Outport
  Sum : Outport  Port=2
  wires:
  Half_Adder1/1(Sum) -> Sum/1
  Carry In/1 -> Half_Adder1/2(y)
  Logical Operator/1 -> Carry/1
  Half_Adder1/2(Carry) -> Logical Operator/1
  A/1 -> Half_Adder/1(x)
  B/1 -> Half_Adder/2(y)
  Half_Adder/2(Carry) -> Logical Operator/2
  Half_Adder/1(Sum) -> Half_Adder1/1(x)

== system labFinal_8/8-Bit_Processor/8-bit_Adder/Concat ==
  S 2^7 : Inport
  S 2^6 : Inport  Port=2
  S 2^5 : Inport  Port=3
  S 2^4 : Inport  Port=4
  S 2^3 : Inport  Port=5
  S 2^2 : Inport  Port=6
  S 2^1 : Inport  Port=7
  S 2^0 : Inport  Port=8
  Bit Concat : hdlsllib/Logic and Bit Operations/Bit Concat  numInputs=8
      settings: SourceProductName=HDL Coder  SourceProductBaseCode=HD
  unsign Int : Outport
  wires:
  Bit Concat/1 -> unsign Int/1
  S 2^3/1 -> Bit Concat/5
  S 2^5/1 -> Bit Concat/3
  S 2^4/1 -> Bit Concat/4
  S 2^0/1 -> Bit Concat/8
  S 2^7/1 -> Bit Concat/1
  S 2^1/1 -> Bit Concat/7
  S 2^6/1 -> Bit Concat/2
  S 2^2/1 -> Bit Concat/6

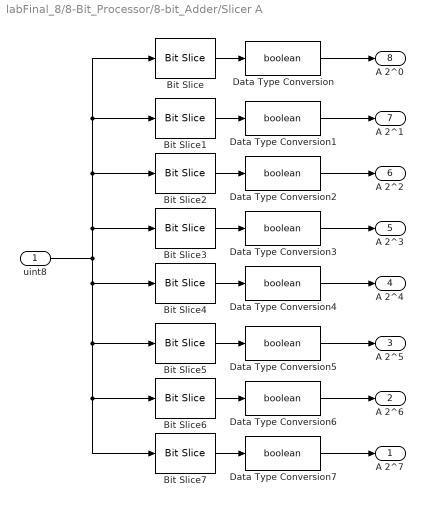
== system labFinal_8/8-Bit_Processor/8-bit_Adder/Slicer A ==
  uint8 : Inport  OutDataTypeStr=uint8  SampleTime=1
  Bit Slice : hdlsllib/Logic and Bit Operations/Bit Slice  lidx=0  ridx=0
  Bit Slice1 : hdlsllib/Logic and Bit Operations/Bit Slice  lidx=1  ridx=1
  Bit Slice2 : hdlsllib/Logic and Bit Operations/Bit Slice  lidx=2  ridx=2
  Bit Slice3 : hdlsllib/Logic and Bit Operations/Bit Slice  lidx=3  ridx=3
  Bit Slice4 : hdlsllib/Logic and Bit Operations/Bit Slice  lidx=4  ridx=4
  Bit Slice5 : hdlsllib/Logic and Bit Operations/Bit Slice  lidx=5  ridx=5
  Bit Slice6 : hdlsllib/Logic and Bit Operations/Bit Slice  lidx=6  ridx=6
  Bit Slice7 : hdlsllib/Logic and Bit Operations/Bit Slice  lidx=7  ridx=7
  Data Type Conversion{,1..7} (8 alike) : DataTypeConversion  OutDataTypeStr=boolean
  A 2^7 : Outport
  A 2^6 : Outport  Port=2
  A 2^5 : Outport  Port=3
  A 2^4 : Outport  Port=4
  A 2^3 : Outport  Port=5
  A 2^2 : Outport  Port=6
  A 2^1 : Outport  Port=7
  "A 2^0 " : Outport  Port=8
  wires:
  Data Type Conversion/1 -> "A 2^0 "/1
  Data Type Conversion5/1 -> A 2^5/1
  Bit Slice1/1 -> Data Type Conversion1/1
  Bit Slice5/1 -> Data Type Conversion5/1
  Bit Slice7/1 -> Data Type Conversion7/1
  Bit Slice2/1 -> Data Type Conversion2/1
  Bit Slice3/1 -> Data Type Conversion3/1
  Data Type Conversion6/1 -> A 2^6/1
  Bit Slice4/1 -> Data Type Conversion4/1
  uint8/1 -> Bit Slice4/1, Bit Slice5/1, Bit Slice6/1, Bit Slice7/1, Bit Slice3/1, Bit Slice2/1, Bit Slice1/1, Bit Slice/1
  Data Type Conversion1/1 -> A 2^1/1
  Data Type Conversion2/1 -> A 2^2/1
  Bit Slice/1 -> Data Type Conversion/1
  Bit Slice6/1 -> Data Type Conversion6/1
  Data Type Conversion3/1 -> A 2^3/1
  Data Type Conversion4/1 -> A 2^4/1
  Data Type Conversion7/1 -> A 2^7/1

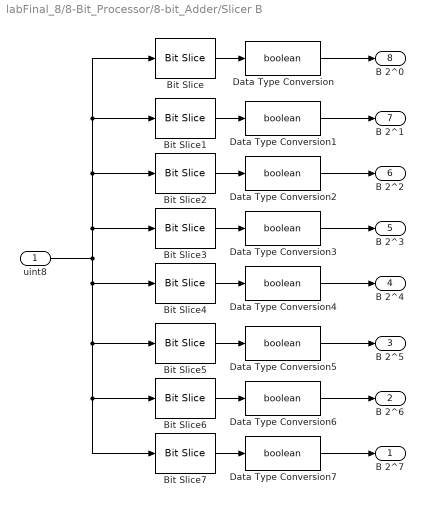
== system labFinal_8/8-Bit_Processor/8-bit_Adder/Slicer B ==
  uint8 : Inport  OutDataTypeStr=uint8  SampleTime=1
  Bit Slice : hdlsllib/Logic and Bit Operations/Bit Slice  lidx=0  ridx=0
  Bit Slice1 : hdlsllib/Logic and Bit Operations/Bit Slice  lidx=1  ridx=1
  Bit Slice2 : hdlsllib/Logic and Bit Operations/Bit Slice  lidx=2  ridx=2
  Bit Slice3 : hdlsllib/Logic and Bit Operations/Bit Slice  lidx=3  ridx=3
  Bit Slice4 : hdlsllib/Logic and Bit Operations/Bit Slice  lidx=4  ridx=4
  Bit Slice5 : hdlsllib/Logic and Bit Operations/Bit Slice  lidx=5  ridx=5
  Bit Slice6 : hdlsllib/Logic and Bit Operations/Bit Slice  lidx=6  ridx=6
  Bit Slice7 : hdlsllib/Logic and Bit Operations/Bit Slice  lidx=7  ridx=7
  Data Type Conversion{,1..7} (8 alike) : DataTypeConversion  OutDataTypeStr=boolean
  B 2^7 : Outport
  B 2^6 : Outport  Port=2
  B 2^5 : Outport  Port=3
  B 2^4 : Outport  Port=4
  B 2^3 : Outport  Port=5
  B 2^2 : Outport  Port=6
  B 2^1 : Outport  Port=7
  "B 2^0 " : Outport  Port=8
  wires:
  Data Type Conversion/1 -> "B 2^0 "/1
  Data Type Conversion5/1 -> B 2^5/1
  Bit Slice1/1 -> Data Type Conversion1/1
  Bit Slice5/1 -> Data Type Conversion5/1
  Bit Slice7/1 -> Data Type Conversion7/1
  Bit Slice2/1 -> Data Type Conversion2/1
  Bit Slice3/1 -> Data Type Conversion3/1
  Data Type Conversion6/1 -> B 2^6/1
  Bit Slice4/1 -> Data Type Conversion4/1
  uint8/1 -> Bit Slice4/1, Bit Slice5/1, Bit Slice6/1, Bit Slice7/1, Bit Slice3/1, Bit Slice2/1, Bit Slice1/1, Bit Slice/1
  Data Type Conversion1/1 -> B 2^1/1
  Data Type Conversion2/1 -> B 2^2/1
  Bit Slice/1 -> Data Type Conversion/1
  Bit Slice6/1 -> Data Type Conversion6/1
  Data Type Conversion3/1 -> B 2^3/1
  Data Type Conversion4/1 -> B 2^4/1
  Data Type Conversion7/1 -> B 2^7/1

== system labFinal_8/8-Bit_Processor/8-bit_Bitwise_AND/Concat ==
  S 2^7 : Inport
  S 2^6 : Inport  Port=2
  S 2^5 : Inport  Port=3
  S 2^4 : Inport  Port=4
  S 2^3 : Inport  Port=5
  S 2^2 : Inport  Port=6
  S 2^1 : Inport  Port=7
  S 2^0 : Inport  Port=8
  Bit Concat : hdlsllib/Logic and Bit Operations/Bit Concat  numInputs=8
      settings: SourceProductName=HDL Coder  SourceProductBaseCode=HD
  unsign Int : Outport
  wires:
  Bit Concat/1 -> unsign Int/1
  S 2^3/1 -> Bit Concat/5
  S 2^5/1 -> Bit Concat/3
  S 2^4/1 -> Bit Concat/4
  S 2^0/1 -> Bit Concat/8
  S 2^7/1 -> Bit Concat/1
  S 2^1/1 -> Bit Concat/7
  S 2^6/1 -> Bit Concat/2
  S 2^2/1 -> Bit Concat/6

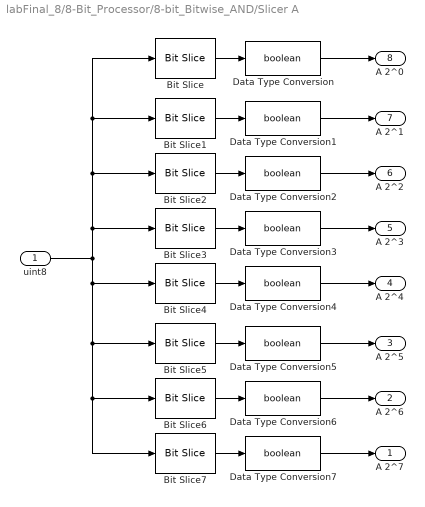
== system labFinal_8/8-Bit_Processor/8-bit_Bitwise_AND/Slicer A ==
  uint8 : Inport  OutDataTypeStr=uint8  SampleTime=1
  Bit Slice : hdlsllib/Logic and Bit Operations/Bit Slice  lidx=0  ridx=0
  Bit Slice1 : hdlsllib/Logic and Bit Operations/Bit Slice  lidx=1  ridx=1
  Bit Slice2 : hdlsllib/Logic and Bit Operations/Bit Slice  lidx=2  ridx=2
  Bit Slice3 : hdlsllib/Logic and Bit Operations/Bit Slice  lidx=3  ridx=3
  Bit Slice4 : hdlsllib/Logic and Bit Operations/Bit Slice  lidx=4  ridx=4
  Bit Slice5 : hdlsllib/Logic and Bit Operations/Bit Slice  lidx=5  ridx=5
  Bit Slice6 : hdlsllib/Logic and Bit Operations/Bit Slice  lidx=6  ridx=6
  Bit Slice7 : hdlsllib/Logic and Bit Operations/Bit Slice  lidx=7  ridx=7
  Data Type Conversion{,1..7} (8 alike) : DataTypeConversion  OutDataTypeStr=boolean
  A 2^7 : Outport
  A 2^6 : Outport  Port=2
  A 2^5 : Outport  Port=3
  A 2^4 : Outport  Port=4
  A 2^3 : Outport  Port=5
  A 2^2 : Outport  Port=6
  A 2^1 : Outport  Port=7
  "A 2^0 " : Outport  Port=8
  wires:
  Data Type Conversion/1 -> "A 2^0 "/1
  Data Type Conversion5/1 -> A 2^5/1
  Bit Slice1/1 -> Data Type Conversion1/1
  Bit Slice5/1 -> Data Type Conversion5/1
  Bit Slice7/1 -> Data Type Conversion7/1
  Bit Slice2/1 -> Data Type Conversion2/1
  Bit Slice3/1 -> Data Type Conversion3/1
  Data Type Conversion6/1 -> A 2^6/1
  Bit Slice4/1 -> Data Type Conversion4/1
  uint8/1 -> Bit Slice4/1, Bit Slice5/1, Bit Slice6/1, Bit Slice7/1, Bit Slice3/1, Bit Slice2/1, Bit Slice1/1, Bit Slice/1
  Data Type Conversion1/1 -> A 2^1/1
  Data Type Conversion2/1 -> A 2^2/1
  Bit Slice/1 -> Data Type Conversion/1
  Bit Slice6/1 -> Data Type Conversion6/1
  Data Type Conversion3/1 -> A 2^3/1
  Data Type Conversion4/1 -> A 2^4/1
  Data Type Conversion7/1 -> A 2^7/1

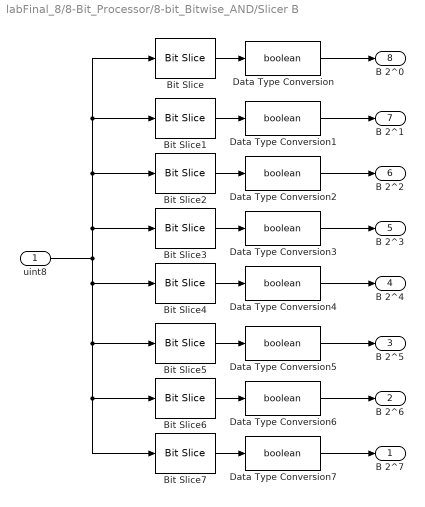
== system labFinal_8/8-Bit_Processor/8-bit_Bitwise_AND/Slicer B ==
  uint8 : Inport  OutDataTypeStr=uint8  SampleTime=1
  Bit Slice : hdlsllib/Logic and Bit Operations/Bit Slice  lidx=0  ridx=0
  Bit Slice1 : hdlsllib/Logic and Bit Operations/Bit Slice  lidx=1  ridx=1
  Bit Slice2 : hdlsllib/Logic and Bit Operations/Bit Slice  lidx=2  ridx=2
  Bit Slice3 : hdlsllib/Logic and Bit Operations/Bit Slice  lidx=3  ridx=3
  Bit Slice4 : hdlsllib/Logic and Bit Operations/Bit Slice  lidx=4  ridx=4
  Bit Slice5 : hdlsllib/Logic and Bit Operations/Bit Slice  lidx=5  ridx=5
  Bit Slice6 : hdlsllib/Logic and Bit Operations/Bit Slice  lidx=6  ridx=6
  Bit Slice7 : hdlsllib/Logic and Bit Operations/Bit Slice  lidx=7  ridx=7
  Data Type Conversion{,1..7} (8 alike) : DataTypeConversion  OutDataTypeStr=boolean
  B 2^7 : Outport
  B 2^6 : Outport  Port=2
  B 2^5 : Outport  Port=3
  B 2^4 : Outport  Port=4
  B 2^3 : Outport  Port=5
  B 2^2 : Outport  Port=6
  B 2^1 : Outport  Port=7
  "B 2^0 " : Outport  Port=8
  wires:
  Data Type Conversion/1 -> "B 2^0 "/1
  Data Type Conversion5/1 -> B 2^5/1
  Bit Slice1/1 -> Data Type Conversion1/1
  Bit Slice5/1 -> Data Type Conversion5/1
  Bit Slice7/1 -> Data Type Conversion7/1
  Bit Slice2/1 -> Data Type Conversion2/1
  Bit Slice3/1 -> Data Type Conversion3/1
  Data Type Conversion6/1 -> B 2^6/1
  Bit Slice4/1 -> Data Type Conversion4/1
  uint8/1 -> Bit Slice4/1, Bit Slice5/1, Bit Slice6/1, Bit Slice7/1, Bit Slice3/1, Bit Slice2/1, Bit Slice1/1, Bit Slice/1
  Data Type Conversion1/1 -> B 2^1/1
  Data Type Conversion2/1 -> B 2^2/1
  Bit Slice/1 -> Data Type Conversion/1
  Bit Slice6/1 -> Data Type Conversion6/1
  Data Type Conversion3/1 -> B 2^3/1
  Data Type Conversion4/1 -> B 2^4/1
  Data Type Conversion7/1 -> B 2^7/1

== system labFinal_8/8-Bit_Processor/8-bit_Multiply/2^1 ==
  A : Inport
  B : Inport  Port=2
  Cin : Inport  Port=3
  Half_Adder : Subsystem
  Half_Adder1 : Subsystem
  Logical Operator : Logic  Operator=OR  AllPortsSameDT=off  OutDataTypeStr=boolean
  C : Outport
  S : Outport  Port=2
  wires:
  Half_Adder1/1(Sum) -> S/1
  Cin/1 -> Half_Adder1/2(y)
  Logical Operator/1 -> C/1
  Half_Adder1/2(Carry) -> Logical Operator/1
  A/1 -> Half_Adder/1(x)
  B/1 -> Half_Adder/2(y)
  Half_Adder/2(Carry) -> Logical Operator/2
  Half_Adder/1(Sum) -> Half_Adder1/1(x)

== system labFinal_8/8-Bit_Processor/8-bit_Multiply/2^10 ==
  A : Inport
  B : Inport  Port=2
  Cin : Inport  Port=3
  Half_Adder : Subsystem
  Half_Adder1 : Subsystem
  Logical Operator : Logic  Operator=OR  AllPortsSameDT=off  OutDataTypeStr=boolean
  C : Outport
  S : Outport  Port=2
  wires:
  Half_Adder1/1(Sum) -> S/1
  Cin/1 -> Half_Adder1/2(y)
  Logical Operator/1 -> C/1
  Half_Adder1/2(Carry) -> Logical Operator/1
  A/1 -> Half_Adder/1(x)
  B/1 -> Half_Adder/2(y)
  Half_Adder/2(Carry) -> Logical Operator/2
  Half_Adder/1(Sum) -> Half_Adder1/1(x)

== system labFinal_8/8-Bit_Processor/8-bit_Multiply/2^11 ==
  A : Inport
  B : Inport  Port=2
  Cin : Inport  Port=3
  Half_Adder : Subsystem
  Half_Adder1 : Subsystem
  Logical Operator : Logic  Operator=OR  AllPortsSameDT=off  OutDataTypeStr=boolean
  C : Outport
  S : Outport  Port=2
  wires:
  Half_Adder1/1(Sum) -> S/1
  Cin/1 -> Half_Adder1/2(y)
  Logical Operator/1 -> C/1
  Half_Adder1/2(Carry) -> Logical Operator/1
  A/1 -> Half_Adder/1(x)
  B/1 -> Half_Adder/2(y)
  Half_Adder/2(Carry) -> Logical Operator/2
  Half_Adder/1(Sum) -> Half_Adder1/1(x)

== system labFinal_8/8-Bit_Processor/8-bit_Multiply/2^12 ==
  A : Inport
  B : Inport  Port=2
  Cin : Inport  Port=3
  Half_Adder : Subsystem
  Half_Adder1 : Subsystem
  Logical Operator : Logic  Operator=OR  AllPortsSameDT=off  OutDataTypeStr=boolean
  C : Outport
  S : Outport  Port=2
  wires:
  Half_Adder1/1(Sum) -> S/1
  Cin/1 -> Half_Adder1/2(y)
  Logical Operator/1 -> C/1
  Half_Adder1/2(Carry) -> Logical Operator/1
  A/1 -> Half_Adder/1(x)
  B/1 -> Half_Adder/2(y)
  Half_Adder/2(Carry) -> Logical Operator/2
  Half_Adder/1(Sum) -> Half_Adder1/1(x)

== system labFinal_8/8-Bit_Processor/8-bit_Multiply/2^13 ==
  A : Inport
  B : Inport  Port=2
  Cin : Inport  Port=3
  Half_Adder : Subsystem
  Half_Adder1 : Subsystem
  Logical Operator : Logic  Operator=OR  AllPortsSameDT=off  OutDataTypeStr=boolean
  C : Outport
  S : Outport  Port=2
  wires:
  Half_Adder1/1(Sum) -> S/1
  Cin/1 -> Half_Adder1/2(y)
  Logical Operator/1 -> C/1
  Half_Adder1/2(Carry) -> Logical Operator/1
  A/1 -> Half_Adder/1(x)
  B/1 -> Half_Adder/2(y)
  Half_Adder/2(Carry) -> Logical Operator/2
  Half_Adder/1(Sum) -> Half_Adder1/1(x)

== system labFinal_8/8-Bit_Processor/8-bit_Multiply/2^14 ==
  A : Inport
  B : Inport  Port=2
  Cin : Inport  Port=3
  Half_Adder : Subsystem
  Half_Adder1 : Subsystem
  Logical Operator : Logic  Operator=OR  AllPortsSameDT=off  OutDataTypeStr=boolean
  C : Outport
  S : Outport  Port=2
  wires:
  Half_Adder1/1(Sum) -> S/1
  Cin/1 -> Half_Adder1/2(y)
  Logical Operator/1 -> C/1
  Half_Adder1/2(Carry) -> Logical Operator/1
  A/1 -> Half_Adder/1(x)
  B/1 -> Half_Adder/2(y)
  Half_Adder/2(Carry) -> Logical Operator/2
  Half_Adder/1(Sum) -> Half_Adder1/1(x)

== system labFinal_8/8-Bit_Processor/8-bit_Multiply/2^15 ==
  A : Inport
  B : Inport  Port=2
  Cin : Inport  Port=3
  Half_Adder : Subsystem
  Half_Adder1 : Subsystem
  Logical Operator : Logic  Operator=OR  AllPortsSameDT=off  OutDataTypeStr=boolean
  C : Outport
  S : Outport  Port=2
  wires:
  Half_Adder1/1(Sum) -> S/1
  Cin/1 -> Half_Adder1/2(y)
  Logical Operator/1 -> C/1
  Half_Adder1/2(Carry) -> Logical Operator/1
  A/1 -> Half_Adder/1(x)
  B/1 -> Half_Adder/2(y)
  Half_Adder/2(Carry) -> Logical Operator/2
  Half_Adder/1(Sum) -> Half_Adder1/1(x)

== system labFinal_8/8-Bit_Processor/8-bit_Multiply/2^16 ==
  A : Inport
  B : Inport  Port=2
  Cin : Inport  Port=3
  Half_Adder : Subsystem
  Half_Adder1 : Subsystem
  Logical Operator : Logic  Operator=OR  AllPortsSameDT=off  OutDataTypeStr=boolean
  C : Outport
  S : Outport  Port=2
  wires:
  Half_Adder1/1(Sum) -> S/1
  Cin/1 -> Half_Adder1/2(y)
  Logical Operator/1 -> C/1
  Half_Adder1/2(Carry) -> Logical Operator/1
  A/1 -> Half_Adder/1(x)
  B/1 -> Half_Adder/2(y)
  Half_Adder/2(Carry) -> Logical Operator/2
  Half_Adder/1(Sum) -> Half_Adder1/1(x)

== system labFinal_8/8-Bit_Processor/8-bit_Multiply/2^17 ==
  A : Inport
  B : Inport  Port=2
  Cin : Inport  Port=3
  Half_Adder : Subsystem
  Half_Adder1 : Subsystem
  Logical Operator : Logic  Operator=OR  AllPortsSameDT=off  OutDataTypeStr=boolean
  C : Outport
  S : Outport  Port=2
  wires:
  Half_Adder1/1(Sum) -> S/1
  Cin/1 -> Half_Adder1/2(y)
  Logical Operator/1 -> C/1
  Half_Adder1/2(Carry) -> Logical Operator/1
  A/1 -> Half_Adder/1(x)
  B/1 -> Half_Adder/2(y)
  Half_Adder/2(Carry) -> Logical Operator/2
  Half_Adder/1(Sum) -> Half_Adder1/1(x)

== system labFinal_8/8-Bit_Processor/8-bit_Multiply/2^18 ==
  A : Inport
  B : Inport  Port=2
  Cin : Inport  Port=3
  Half_Adder : Subsystem
  Half_Adder1 : Subsystem
  Logical Operator : Logic  Operator=OR  AllPortsSameDT=off  OutDataTypeStr=boolean
  C : Outport
  S : Outport  Port=2
  wires:
  Half_Adder1/1(Sum) -> S/1
  Cin/1 -> Half_Adder1/2(y)
  Logical Operator/1 -> C/1
  Half_Adder1/2(Carry) -> Logical Operator/1
  A/1 -> Half_Adder/1(x)
  B/1 -> Half_Adder/2(y)
  Half_Adder/2(Carry) -> Logical Operator/2
  Half_Adder/1(Sum) -> Half_Adder1/1(x)

== system labFinal_8/8-Bit_Processor/8-bit_Multiply/2^19 ==
  A : Inport
  B : Inport  Port=2
  Cin : Inport  Port=3
  Half_Adder : Subsystem
  Half_Adder1 : Subsystem
  Logical Operator : Logic  Operator=OR  AllPortsSameDT=off  OutDataTypeStr=boolean
  C : Outport
  S : Outport  Port=2
  wires:
  Half_Adder1/1(Sum) -> S/1
  Cin/1 -> Half_Adder1/2(y)
  Logical Operator/1 -> C/1
  Half_Adder1/2(Carry) -> Logical Operator/1
  A/1 -> Half_Adder/1(x)
  B/1 -> Half_Adder/2(y)
  Half_Adder/2(Carry) -> Logical Operator/2
  Half_Adder/1(Sum) -> Half_Adder1/1(x)
